simulink model "FirstPress"  (R2022b)
settings: Solver=FixedStepAuto  StartTime=0.0  StopTime=10.0  FixedStep=0.08  RelTol=1e-3
model workspace (MAT data in the model file):
  ContractValidatorBlocksMap = containers.Map
  ContractValidatorBlocksMap.serialization.keys = {'FirstPass/Req_s3_1_2_2_p19_2/validator', 'FirstPass/Req_s3_1_2_2_p19_3/validator', 'FirstPass/contract/validator', 'FirstPass/contract1/validator'}
  ContractValidatorBlocksMap.serialization.values{1}.block = 'FirstPass/Req_s3_1_2_2_p19_2/validator'
  ContractValidatorBlocksMap.serialization.values{1}.assumePorts = 0
  ContractValidatorBlocksMap.serialization.values{1}.guaranteePorts = 1
  ContractValidatorBlocksMap.serialization.values{1}.modeBlocksPorts = 0
  ContractValidatorBlocksMap.serialization.values{1}.portHandles.Inport = 2748.11108398
  ContractValidatorBlocksMap.serialization.values{1}.portHandles.Outport = 2749.11108398
  ContractValidatorBlocksMap.serialization.values{1}.portHandles.Enable = []
  ContractValidatorBlocksMap.serialization.values{1}.portHandles.Trigger = []
  ContractValidatorBlocksMap.serialization.values{1}.portHandles.State = []
  ContractValidatorBlocksMap.serialization.values{1}.portHandles.LConn = []
  ContractValidatorBlocksMap.serialization.values{1}.portHandles.RConn = []
  ContractValidatorBlocksMap.serialization.values{1}.portHandles.Ifaction = []
  ContractValidatorBlocksMap.serialization.values{1}.portHandles.Reset = []
  ContractValidatorBlocksMap.serialization.values{1}.portConnectivity(1).Type = '1'
  ContractValidatorBlocksMap.serialization.values{1}.portConnectivity(1).Position = [365 90]
  ContractValidatorBlocksMap.serialization.values{1}.portConnectivity(1).SrcBlock = 2685.11108398
  ContractValidatorBlocksMap.serialization.values{1}.portConnectivity(1).SrcPort = 0
  ContractValidatorBlocksMap.serialization.values{1}.portConnectivity(1).DstBlock = []
  ContractValidatorBlocksMap.serialization.values{1}.portConnectivity(1).DstPort = []
  ContractValidatorBlocksMap.serialization.values{1}.portConnectivity(2).Type = '1'
  ContractValidatorBlocksMap.serialization.values{1}.portConnectivity(2).Position = [500 90]
  ContractValidatorBlocksMap.serialization.values{1}.portConnectivity(2).SrcBlock = []
  ContractValidatorBlocksMap.serialization.values{1}.portConnectivity(2).SrcPort = []
  ContractValidatorBlocksMap.serialization.values{1}.portConnectivity(2).DstBlock = 2694.11108398
  ContractValidatorBlocksMap.serialization.values{1}.portConnectivity(2).DstPort = 0
  ContractValidatorBlocksMap.serialization.values{2}.block = 'FirstPass/Req_s3_1_2_2_p19_3/validator'
  ContractValidatorBlocksMap.serialization.values{2}.assumePorts = 0
  ContractValidatorBlocksMap.serialization.values{2}.guaranteePorts = 1
  ContractValidatorBlocksMap.serialization.values{2}.modeBlocksPorts = 0
  ContractValidatorBlocksMap.serialization.values{2}.portHandles.Inport = 2746.11132812
  ContractValidatorBlocksMap.serialization.values{2}.portHandles.Outport = 2747.11108398
  ContractValidatorBlocksMap.serialization.values{2}.portHandles.Enable = []
  ContractValidatorBlocksMap.serialization.values{2}.portHandles.Trigger = []
  ContractValidatorBlocksMap.serialization.values{2}.portHandles.State = []
  ContractValidatorBlocksMap.serialization.values{2}.portHandles.LConn = []
  ContractValidatorBlocksMap.serialization.values{2}.portHandles.RConn = []
  ContractValidatorBlocksMap.serialization.values{2}.portHandles.Ifaction = []
  ContractValidatorBlocksMap.serialization.values{2}.portHandles.Reset = []
  ContractValidatorBlocksMap.serialization.values{2}.portConnectivity(1).Type = '1'
  ContractValidatorBlocksMap.serialization.values{2}.portConnectivity(1).Position = [365 75]
  ContractValidatorBlocksMap.serialization.values{2}.portConnectivity(1).SrcBlock = 2703.11108398
  ContractValidatorBlocksMap.serialization.values{2}.portConnectivity(1).SrcPort = 0
  ContractValidatorBlocksMap.serialization.values{2}.portConnectivity(1).DstBlock = []
  ContractValidatorBlocksMap.serialization.values{2}.portConnectivity(1).DstPort = []
  ContractValidatorBlocksMap.serialization.values{2}.portConnectivity(2).Type = '1'
  ContractValidatorBlocksMap.serialization.values{2}.portConnectivity(2).Position = [500 75]
  ContractValidatorBlocksMap.serialization.values{2}.portConnectivity(2).SrcBlock = []
  ContractValidatorBlocksMap.serialization.values{2}.portConnectivity(2).SrcPort = []
  ContractValidatorBlocksMap.serialization.values{2}.portConnectivity(2).DstBlock = 2720.11108398
  ContractValidatorBlocksMap.serialization.values{2}.portConnectivity(2).DstPort = 0
  ContractValidatorBlocksMap.serialization.values{3}.block = 'FirstPass/contract/validator'
  ContractValidatorBlocksMap.serialization.values{3}.assumePorts = 0
  ContractValidatorBlocksMap.serialization.values{3}.guaranteePorts = 1
  ContractValidatorBlocksMap.serialization.values{3}.modeBlocksPorts = 0
  ContractValidatorBlocksMap.serialization.values{3}.portHandles.Inport = 1491.35229492
  ContractValidatorBlocksMap.serialization.values{3}.portHandles.Outport = 1492.35205078
  ContractValidatorBlocksMap.serialization.values{3}.portHandles.Enable = []
  ContractValidatorBlocksMap.serialization.values{3}.portHandles.Trigger = []
  ContractValidatorBlocksMap.serialization.values{3}.portHandles.State = []
  ContractValidatorBlocksMap.serialization.values{3}.portHandles.LConn = []
  ContractValidatorBlocksMap.serialization.values{3}.portHandles.RConn = []
  ContractValidatorBlocksMap.serialization.values{3}.portHandles.Ifaction = []
  ContractValidatorBlocksMap.serialization.values{3}.portHandles.Reset = []
  ContractValidatorBlocksMap.serialization.values{3}.portConnectivity(1).Type = '1'
  ContractValidatorBlocksMap.serialization.values{3}.portConnectivity(1).Position = [365 75]
  ContractValidatorBlocksMap.serialization.values{3}.portConnectivity(1).SrcBlock = 1448.35205078
  ContractValidatorBlocksMap.serialization.values{3}.portConnectivity(1).SrcPort = 0
  ContractValidatorBlocksMap.serialization.values{3}.portConnectivity(1).DstBlock = []
  ContractValidatorBlocksMap.serialization.values{3}.portConnectivity(1).DstPort = []
  ContractValidatorBlocksMap.serialization.values{3}.portConnectivity(2).Type = '1'
  ContractValidatorBlocksMap.serialization.values{3}.portConnectivity(2).Position = [500 75]
  ContractValidatorBlocksMap.serialization.values{3}.portConnectivity(2).SrcBlock = []
  ContractValidatorBlocksMap.serialization.values{3}.portConnectivity(2).SrcPort = []
  ContractValidatorBlocksMap.serialization.values{3}.portConnectivity(2).DstBlock = 1465.35205078
  ContractValidatorBlocksMap.serialization.values{3}.portConnectivity(2).DstPort = 0
  ContractValidatorBlocksMap.serialization.values{4}.block = 'FirstPass/contract1/validator'
  ContractValidatorBlocksMap.serialization.values{4}.assumePorts = 0
  ContractValidatorBlocksMap.serialization.values{4}.guaranteePorts = 1
  ContractValidatorBlocksMap.serialization.values{4}.modeBlocksPorts = 0
  ContractValidatorBlocksMap.serialization.values{4}.portHandles.Inport = 5485.11975098
  ContractValidatorBlocksMap.serialization.values{4}.portHandles.Outport = 5486.11975098
  ContractValidatorBlocksMap.serialization.values{4}.portHandles.Enable = []
  ContractValidatorBlocksMap.serialization.values{4}.portHandles.Trigger = []
  ContractValidatorBlocksMap.serialization.values{4}.portHandles.State = []
  ContractValidatorBlocksMap.serialization.values{4}.portHandles.LConn = []
  ContractValidatorBlocksMap.serialization.values{4}.portHandles.RConn = []
  ContractValidatorBlocksMap.serialization.values{4}.portHandles.Ifaction = []
  ContractValidatorBlocksMap.serialization.values{4}.portHandles.Reset = []
  ContractValidatorBlocksMap.serialization.values{4}.portConnectivity(1).Type = '1'
  ContractValidatorBlocksMap.serialization.values{4}.portConnectivity(1).Position = [365 75]
  ContractValidatorBlocksMap.serialization.values{4}.portConnectivity(1).SrcBlock = 5292.11987305
  ContractValidatorBlocksMap.serialization.values{4}.portConnectivity(1).SrcPort = 0
  ContractValidatorBlocksMap.serialization.values{4}.portConnectivity(1).DstBlock = []
  ContractValidatorBlocksMap.serialization.values{4}.portConnectivity(1).DstPort = []
  ContractValidatorBlocksMap.serialization.values{4}.portConnectivity(2).Type = '1'
  ContractValidatorBlocksMap.serialization.values{4}.portConnectivity(2).Position = [500 75]
  ContractValidatorBlocksMap.serialization.values{4}.portConnectivity(2).SrcBlock = []
  ContractValidatorBlocksMap.serialization.values{4}.portConnectivity(2).SrcPort = []
  ContractValidatorBlocksMap.serialization.values{4}.portConnectivity(2).DstBlock = 5462.12011719
  ContractValidatorBlocksMap.serialization.values{4}.portConnectivity(2).DstPort = 0
  ContractValidatorBlocksMap.serialization.uniformity = 0
  ContractValidatorBlocksMap.serialization.keyType = 'char'
  ContractValidatorBlocksMap.serialization.valueType = 'any'
settings Model: Creator=hbourbou  LastModifiedBy=yuzehong
settings SolverCC: AlgebraicLoopSolver=TrustRegion
settings DataIOCC: ReturnWorkspaceOutputs=off
settings OptimizationCC: DefaultParameterBehavior=Inlined  ReuseModelBlockBuffer=on  EnhancedBackFolding=on  PassReuseOutputArgsAs=Individual arguments  OptimizeBlockOrder=speed  DifferentSizesBufferReuse=on  OptimizationCustomize=off  EfficientTunableParamExpr=on
settings DebuggingCC: ParameterTunabilityLossMsg=error  UnconnectedInputMsg=warning  UnconnectedOutputMsg=warning  UnconnectedLineMsg=warning  ArithmeticOperatorsInVariantConditions=warning
settings ModelReferenceCC: EnableRefExpFcnMdlSchedulingChecks=on
settings SFSimCC: SimUseLocalCustomCode=off  MATLABDynamicMemAlloc=off  CustomCodeUndefinedFunction=UseInterfaceOnly
settings RTWCC: Description=Embedded Coder  SystemTargetFile=ert.tlc  GenCodeOnly=on  TemplateMakefile=ert_default_tmf  RTWUseLocalCustomCode=off
settings CodeAppCC: GenerateComments=off  IgnoreCustomStorageClasses=off  OperatorAnnotations=on  SimulinkDataObjDesc=on  SFDataObjDesc=on  SimulinkBlockComments=off
settings ERTTargetCC: TargetLangStandard=C99 (ISO)  GenerateSampleERTMain=on  CodeInterfacePackaging=Reusable function  InlinedParameterPlacement=NonHierarchical  ERTCustomFileTemplate=example_file_process.tlc

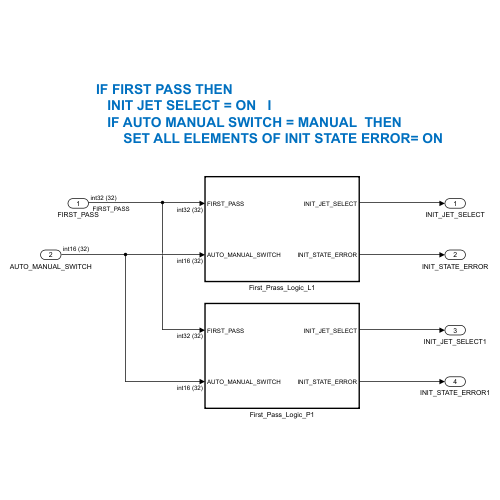
[thumbnail: Simulink's stored preview of the top-level diagram]
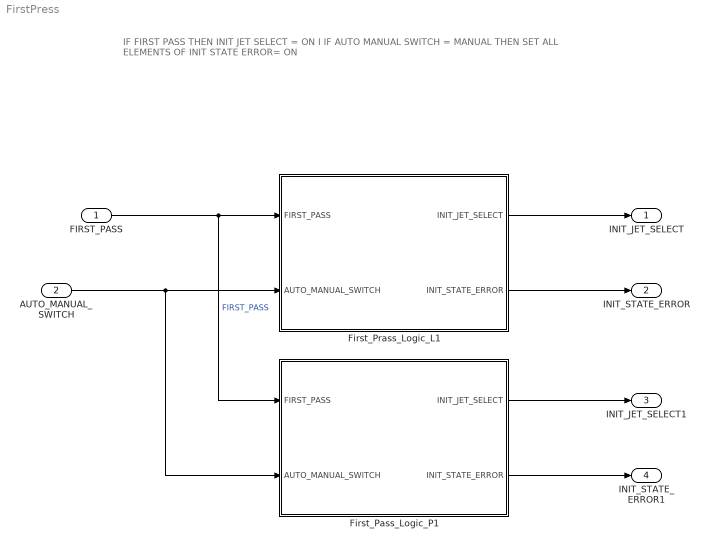
== system FirstPress ==
  note: IF FIRST PASS THEN
      | INIT JET SELECT = ON I
      | IF AUTO MANUAL SWITCH = MANUAL THEN
      | SET ALL ELEMENTS OF INIT STATE ERROR= ON
  FIRST_PASS : Inport  OutDataTypeStr=int32  PortDimensions=32
  AUTO_MANUAL_SWITCH : Inport  Port=2  OutDataTypeStr=int16  PortDimensions=32
  First_Pass_Logic_P1 : Subsystem  TreatAsAtomicUnit=on
      settings: RTWFcnNameOpts=Use subsystem name
  First_Prass_Logic_L1 : Subsystem  TreatAsAtomicUnit=on
      settings: RTWFcnNameOpts=Use subsystem name
  INIT_JET_SELECT : Outport  VectorParamsAs1DForOutWhenUnconnected=off
  INIT_STATE_ERROR : Outport  Port=2  VectorParamsAs1DForOutWhenUnconnected=off
  INIT_JET_SELECT1 : Outport  Port=3  VectorParamsAs1DForOutWhenUnconnected=off
  INIT_STATE_ERROR1 : Outport  Port=4  VectorParamsAs1DForOutWhenUnconnected=off
  wires:
  FIRST_PASS/1 -> First_Pass_Logic_P1/1(FIRST_PASS), First_Prass_Logic_L1/1(FIRST_PASS)  "FIRST_PASS"
  AUTO_MANUAL_SWITCH/1 -> First_Pass_Logic_P1/2(AUTO_MANUAL_SWITCH), First_Prass_Logic_L1/2(AUTO_MANUAL_SWITCH)
  First_Prass_Logic_L1/1(INIT_JET_SELECT) -> INIT_JET_SELECT/1
  First_Prass_Logic_L1/2(INIT_STATE_ERROR) -> INIT_STATE_ERROR/1
  First_Pass_Logic_P1/1(INIT_JET_SELECT) -> INIT_JET_SELECT1/1
  First_Pass_Logic_P1/2(INIT_STATE_ERROR) -> INIT_STATE_ERROR1/1

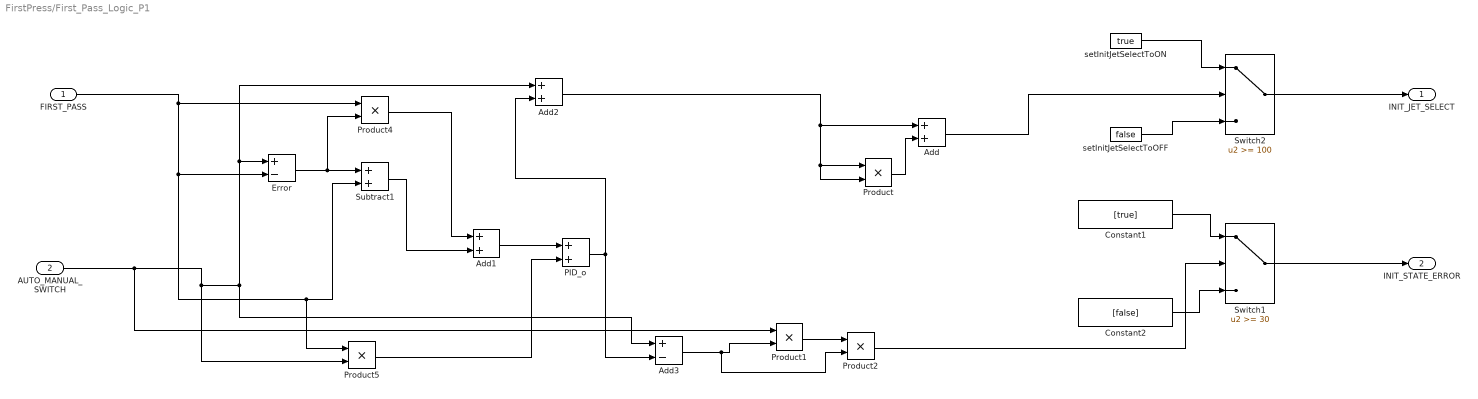
== system FirstPress/First_Pass_Logic_P1 ==
  FIRST_PASS : Inport  OutDataTypeStr=int32  PortDimensions=32
  AUTO_MANUAL_SWITCH : Inport  Port=2  OutDataTypeStr=int16  PortDimensions=32
  Add : Sum  AccumDataTypeStr=int32  SaturateOnIntegerOverflow=on
  Add1 : Sum  OutDataTypeStr=int32  SaturateOnIntegerOverflow=on
  Add2 : Sum  OutDataTypeStr=int32  SaturateOnIntegerOverflow=on
  Add3 : Sum  Inputs=+-  OutDataTypeStr=int32
  Constant1 : Constant  Value=[true]  OutDataTypeStr=boolean
  Constant2 : Constant  Value=[false]  OutDataTypeStr=boolean
  Error : Sum  Inputs=+-  OutDataTypeStr=int32  SaturateOnIntegerOverflow=on
  PID_o : Sum  OutDataTypeStr=int32  SaturateOnIntegerOverflow=on
  Product{,1..2,4..5} (5 alike) : Product  OutDataTypeStr=int32
  Subtract1 : Sum  OutDataTypeStr=int32  SaturateOnIntegerOverflow=on
  Switch1 : Switch  Threshold=30  SaturateOnIntegerOverflow=off  InputSameDT=off
  Switch2 : Switch  Threshold=100  SaturateOnIntegerOverflow=off  InputSameDT=off
  setInitJetSelectToOFF : Constant  Value=false  OutDataTypeStr=boolean
  setInitJetSelectToON : Constant  Value=true  OutDataTypeStr=boolean
  INIT_JET_SELECT : Outport  VectorParamsAs1DForOutWhenUnconnected=off
  INIT_STATE_ERROR : Outport  Port=2  VectorParamsAs1DForOutWhenUnconnected=off
  wires:
  Constant1/1 -> Switch1/1
  Switch1/1 -> INIT_STATE_ERROR/1
  Constant2/1 -> Switch1/3
  Switch2/1 -> INIT_JET_SELECT/1
  setInitJetSelectToON/1 -> Switch2/1
  setInitJetSelectToOFF/1 -> Switch2/3
  PID_o/1 -> Add3/2, Add2/2
  Subtract1/1 -> Add1/2
  Product5/1 -> PID_o/2
  Product4/1 -> Add1/1
  Add1/1 -> PID_o/1
  Error/1 -> Product4/2, Subtract1/1
  FIRST_PASS/1 -> Product5/1, Subtract1/2, Error/2, Product4/1
  AUTO_MANUAL_SWITCH/1 -> Product1/1, Product5/2, Add2/1, Error/1, Add3/1
  Add2/1 -> Add/1, Product/2, Product/1
  Product/1 -> Add/2
  Add/1 -> Switch2/2
  Product1/1 -> Product2/1
  Add3/1 -> Product2/2, Product1/2
  Product2/1 -> Switch1/2

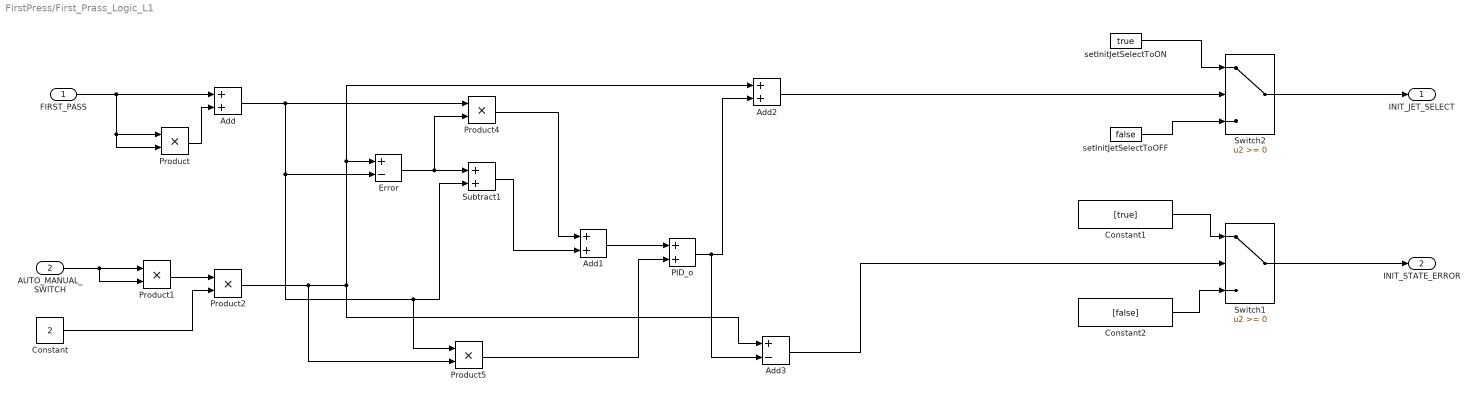
== system FirstPress/First_Prass_Logic_L1 ==
  FIRST_PASS : Inport  OutDataTypeStr=int32  PortDimensions=32
  AUTO_MANUAL_SWITCH : Inport  Port=2  OutDataTypeStr=int16  PortDimensions=32
  Add : Sum  AccumDataTypeStr=int32  SaturateOnIntegerOverflow=on
  Add1 : Sum  OutDataTypeStr=int32  SaturateOnIntegerOverflow=on
  Add2 : Sum  OutDataTypeStr=int32  SaturateOnIntegerOverflow=on
  Add3 : Sum  Inputs=+-  OutDataTypeStr=int32
  Constant : Constant  Value=2  OutDataTypeStr=int32
  Constant1 : Constant  Value=[true]  OutDataTypeStr=boolean
  Constant2 : Constant  Value=[false]  OutDataTypeStr=boolean
  Error : Sum  Inputs=+-  OutDataTypeStr=int32  SaturateOnIntegerOverflow=on
  PID_o : Sum  OutDataTypeStr=int32  SaturateOnIntegerOverflow=on
  Product : Product  OutDataTypeStr=int32
  Product1 : Product
  Product2 : Product  OutDataTypeStr=int32  SaturateOnIntegerOverflow=on
  Product4 : Product  OutDataTypeStr=int32
  Product5 : Product  OutDataTypeStr=int32
  Subtract1 : Sum  OutDataTypeStr=int32  SaturateOnIntegerOverflow=on
  Switch1 : Switch  SaturateOnIntegerOverflow=off  InputSameDT=off
  Switch2 : Switch  SaturateOnIntegerOverflow=off  InputSameDT=off
  setInitJetSelectToOFF : Constant  Value=false  OutDataTypeStr=boolean
  setInitJetSelectToON : Constant  Value=true  OutDataTypeStr=boolean
  INIT_JET_SELECT : Outport  VectorParamsAs1DForOutWhenUnconnected=off
  INIT_STATE_ERROR : Outport  Port=2  VectorParamsAs1DForOutWhenUnconnected=off
  wires:
  Constant1/1 -> Switch1/1
  Switch1/1 -> INIT_STATE_ERROR/1
  Constant2/1 -> Switch1/3
  Switch2/1 -> INIT_JET_SELECT/1
  setInitJetSelectToON/1 -> Switch2/1
  setInitJetSelectToOFF/1 -> Switch2/3
  AUTO_MANUAL_SWITCH/1 -> Product1/2, Product1/1
  FIRST_PASS/1 -> Add/1, Product/2, Product/1
  Product/1 -> Add/2
  Product1/1 -> Product2/1
  Constant/1 -> Product2/2
  PID_o/1 -> Add3/2, Add2/2
  Subtract1/1 -> Add1/2
  Product5/1 -> PID_o/2
  Product4/1 -> Add1/1
  Add2/1 -> Switch2/2
  Add1/1 -> PID_o/1
  Error/1 -> Product4/2, Subtract1/1
  Add/1 -> Product5/1, Subtract1/2, Error/2, Product4/1
  Product2/1 -> Product5/2, Add2/1, Error/1, Add3/1
  Add3/1 -> Switch1/2
